simulink model "Heading_Mode"  (R2016a)
settings: Solver=FixedStepDiscrete  SolverMode=SingleTasking  StartTime=0.0  StopTime=25  FixedStep=1/40  RelTol=1e-3
model workspace (MAT data in the model file):
  hdgGain = Simulink.Parameter
  hdgGain.Value = 0.015
  hdgGain.DataType = 'auto'
  hdgGain.Dimensions = [1 1]
libraries: AP_Lib x1, simulink x1
settings Model: RequirementInfo={} %GIDa_fe9045fd_0412_4b6e_8206_617cc20e6fde  TunableVars=hdgGain  TunableVarsStorageClass=Auto  ParameterArgumentNames=hdgGain  Creator=bpotter  LastModifiedBy=ceren.gebizli
settings DataIOCC: ExternalInput=apin  LoadExternalInput=on  SaveFormat=StructureWithTime  SignalLoggingSaveFormat=ModelDataLogs  DSMLogging=off  SignalLoggingName=Heading_Mode_logsout
settings OptimizationCC: BlockReduction=off  DefaultParameterBehavior=Inlined  InlineInvariantSignals=on  ExpressionDepthLimit=2147483647  EfficientFloat2IntCast=on  EfficientMapNaN2IntZero=off  OptimizeModelRefInitCode=on  MaxStackSize=inf
settings DebuggingCC: SignalInfNanChecking=error  SignalRangeChecking=error  ReadBeforeWriteMsg=EnableAllAsError  WriteAfterWriteMsg=EnableAllAsError  WriteAfterReadMsg=EnableAllAsError  AlgebraicLoopMsg=error  ArtificialAlgebraicLoopMsg=error  SaveWithDisabledLinksMsg=error  SaveWithParameterizedLinksMsg=error  CheckExecutionContextPreStartOutputMsg=on  CheckExecutionContextRuntimeOutputMsg=on  BlockPriorityViolationMsg=error  MaxConsecutiveZCsMsg=warning  SolverPrmCheckMsg=error  InheritedTsInSrcMsg=error  SingleTaskRateTransMsg=error  TasksWithSamePriorityMsg=error  SigSpecEnsureSampleTimeMsg=error  CheckMatrixSingularityMsg=error  IntegerOverflowMsg=error  ParameterUnderflowMsg=error  ParameterPrecisionLossMsg=error  ParameterTunabilityLossMsg=error  UnderSpecifiedDataTypeMsg=error  UnnecessaryDatatypeConvMsg=warning  VectorMatrixConversionMsg=error  SignalLabelMismatchMsg=error  UnconnectedInputMsg=error  UnconnectedOutputMsg=error  UnconnectedLineMsg=error  SFcnCompatibilityMsg=error  UniqueDataStoreMsg=error  BusObjectLabelMismatch=error  RootOutportRequireBusObject=error  AssertControl=DisableAll  ModelReferenceIOMsg=error  ModelReferenceIOMismatchMessage=error  UnknownTsInhSupMsg=error  ModelReferenceDataLoggingMessage=error  ModelReferenceExtraNoncontSigs=none  StateNameClashWarn=warning  StrictBusMsg=ErrorOnBusTreatedAsVector  NonBusSignalsTreatedAsBus=error  IntegerSaturationMsg=error
settings HardwareCC: ProdBitPerPointer=32  ProdLargestAtomicFloat=None  ProdEndianess=BigEndian  ProdWordSize=32  ProdHWDeviceType=32-bit Embedded Processor  TargetHWDeviceType=32-bit Generic
settings ModelReferenceCC: PropagateSignalLabelsOutOfModel=off
settings RTWCC: SystemTargetFile=ert.tlc  TemplateMakefile=ert_default_tmf  GenerateReport=on  RTWVerbose=off  IncludeHyperlinkInReport=on  LaunchReport=on  PortableWordSizes=on  GenerateTraceInfo=on  GenerateTraceReport=on  GenerateTraceReportSl=on  GenerateTraceReportSf=on  GenerateTraceReportEml=on
settings CodeAppCC: ForceParamTrailComments=on  IgnoreCustomStorageClasses=off  MaxIdLength=63  MangleLength=4  CustomSymbolStrType=$N$R$M  InternalIdentifier=Classic  ReqsInCode=on
settings ERTTargetCC: UtilityFuncGeneration=Shared location  GenerateSampleERTMain=on  IncludeMdlTerminateFcn=off  GeneratePreprocessorConditionals=Disable all  SuppressErrorStatus=on  SupportAbsoluteTime=off  SupportNonFinite=off  SupportComplex=off  ParenthesesLevel=Maximum  InlinedParameterPlacement=NonHierarchical  MultiInstanceErrorCode=None  ERTCustomFileTemplate=example_file_process.tlc  PreserveExpressionOrder=on  PreserveIfCondition=on  ConvertIfToSwitch=off  SuppressUnreachableDefaultCases=off
settings ConfigComp: CovSaveName=covdata_rollAP  CovMetricSettings=dcmtrzoiwe  CovHTMLOptions=-sRT=1 -aTS=1 -bRG=1 -bTC=1 -hTR=1 -nFC=0 -scm=1 -bcm=1 -xEv=0  CovHtmlReporting=off  CovSaveSingleToWorkspaceVar=off  CovCumulativeVarName=covCumulativeData_rollAP  CovCumulativeReport=on  CovReportOnPause=off

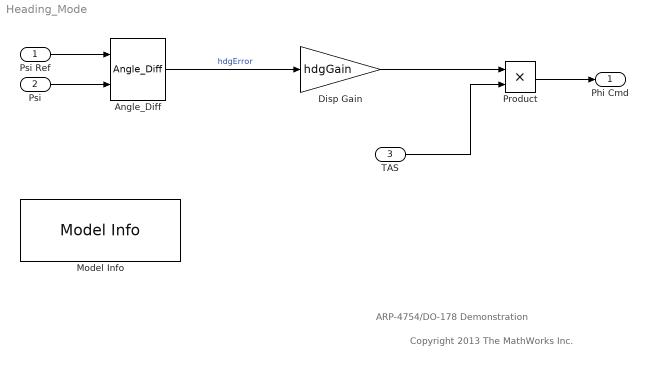
== system Heading_Mode ==
  note: Copyright 2013 The MathWorks Inc.
  note: ARP-4754/DO-178 Demonstration
  Psi Ref : Inport  RequirementInfo="{'other' 'do178b_autopilot_requirements.docx' '@Simulink_requirement_item_10' 'true' '1.10. Heading Performance    ' ' ' ; 'other' 'do178b_autopilot_requirements.docx' '@Simulink_requirement_item_9' 'true' '1.9. Heading Hold Reference' '' } %GIDa_7dc03c75_5e34_4e08_bb6f_6d840def0f56"  OutDataTypeStr=double  PortDimensions=1  SampleTime=1/40  Interpolate=off
  Psi : Inport  RequirementInfo="{'other' 'do178b_autopilot_requirements.docx' '@Simulink_requirement_item_10' 'true' '1.10. Heading Performance     ' '' } %GIDa_4169e82d_42c5_44c7_a191_9b5ca9dcb70a"  Port=2  OutDataTypeStr=double  PortDimensions=1  SampleTime=1/40  Interpolate=off
  TAS : Inport  RequirementInfo="{'other' 'do178b_autopilot_requirements.docx' '@Simulink_requirement_item_10' 'true' '1.10. Heading Performance        ' '' } %GIDa_f893e673_5937_4a6a_88ec_5c2959f3360e"  Port=3  OutDataTypeStr=double  PortDimensions=1  SampleTime=1/40  Interpolate=off
  Angle_Diff : AP_Lib/Angle_Diff
      settings: AttributesFormatString=-180 deg to +180 deg range
  Disp Gain : Gain  RequirementInfo="{'other' 'do178b_autopilot_requirements.docx' '@Simulink_requirement_item_10' 'true' '1.10. Heading Performance       ' '' } %GIDa_e43ec5f2_7e00_48d9_b3be_d6b2fb8df9a5"  Gain=hdgGain
  Model Info : simulink/Model-Wide Utilities/Model Info  BlockCM=none  Frame=on  DisplayStringWithTags=|  HorizontalTextAlignment=Left  LeftAlignmentValue=0.02  SourceBlockDiagram=Heading_Mode  TagMaxNumber=20
      | Heading Mode
      | Author: %<LastModifiedBy>
      | Version: %<ModelVersion>
      | Date: %<LastModificationDate>
  Product : Product  RequirementInfo="{'other' 'do178b_autopilot_requirements.docx' '@Simulink_requirement_item_10' 'true' '1.10. Heading Performance         ' '' } %GIDa_ab0fdff5_b5b7_4090_bee6_e4de829092e0"  RndMeth=Zero
  Phi Cmd : Outport  RequirementInfo="{'other' 'do178b_autopilot_requirements.docx' '@Simulink_requirement_item_10' 'true' '1.10. Heading Performance          ' '' } %GIDa_b1e9aa33_d2c6_47b6_aeae_2214d48474ed"  OutDataTypeStr=double  PortDimensions=1  SampleTime=1/40
  wires:
  Product/1 -> Phi Cmd/1
  Disp Gain/1 -> Product/1
  Angle_Diff/1 -> Disp Gain/1  "hdgError"
  Psi Ref/1 -> Angle_Diff/1
  TAS/1 -> Product/2
  Psi/1 -> Angle_Diff/2
